simulink model "Trac_Energy_Analysis_Final"  (R2018a)
settings: Solver=VariableStepAuto  StartTime=0.0  StopTime=1220  RelTol=1e-3
libraries: qss_tb_library x2, simulink x1
settings Model: Creator=egp  LastModifiedBy=egp

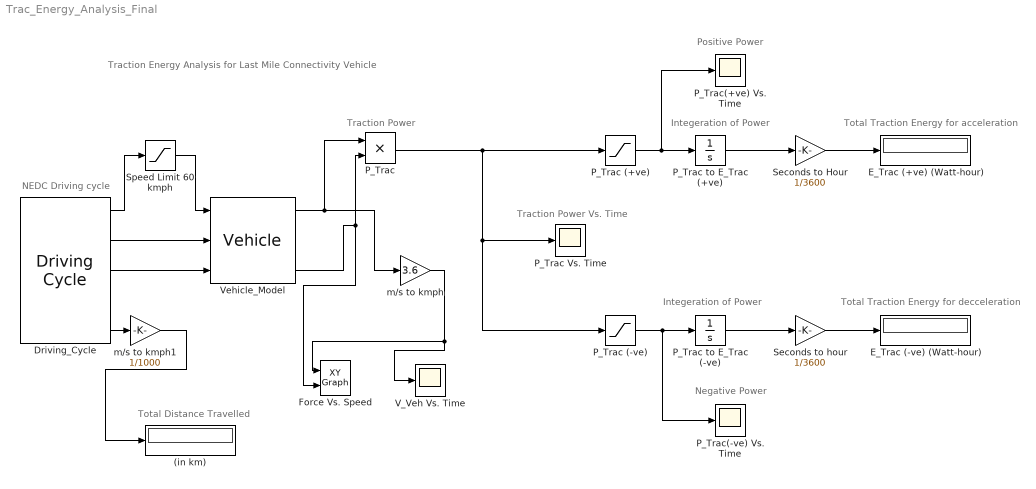
== system Trac_Energy_Analysis_Final ==
  note: Traction Energy Analysis for Last Mile Connectivity Vehicle
  note: Traction Power
  note: NEDC Driving cycle
  note: Total Distance Travelled
  note: Traction Power Vs. Time
  note: Total Traction Energy for acceleration
  note: Total Traction Energy for decceleration
  note: Positive Power
  note: Negative Power
  note: Integeration of Power
  note: Integeration of Power
  (in km) : Display
  Driving_Cycle : qss_tb_library/Driving Cycle/Driving Cycle  Tag=cycle  cyclename1=NEDC  stepsize=1  autostop=on
  E_Trac (+ve) (Watt-hour) : Display
  E_Trac (-ve) (Watt-hour) : Display
  Force Vs. Speed : simulink/Sinks/XY Graph  xmin=0  xmax=65  ymin=-2500  ymax=2500  st=-1
  P_Trac : Product
  P_Trac (+ve) : Saturate  UpperLimit=60000  LowerLimit=0  OutMin=0  OutMax=60000
  P_Trac (-ve) : Saturate  UpperLimit=0  LowerLimit=-60000  OutMin=-60000  OutMax=0
  P_Trac Vs. Time : Scope
  P_Trac to E_Trac (+ve) : Integrator
  P_Trac to E_Trac (-ve) : Integrator
  P_Trac(+ve) Vs. Time : Scope
  P_Trac(-ve) Vs. Time : Scope
  Seconds to Hour : Gain  Gain=1/3600
  Seconds to hour : Gain  Gain=1/3600
  Speed Limit 60 kmph : Saturate  UpperLimit=60/3.6  LowerLimit=0  OutMin=0  OutMax=60/3.6
  V_Veh Vs. Time : Scope
  Vehicle_Model : qss_tb_library/Vehicle/Vehicle  Tag=vehicle  m_f=1750  A_f=2.88  cw=0.5  mu=0.01  k_inertia=5
  m/s to kmph : Gain  Gain=3.6
  m/s to kmph1 : Gain  Gain=1/1000
  wires:
  Driving_Cycle/2 -> Vehicle_Model/2
  Driving_Cycle/3 -> Vehicle_Model/3
  Vehicle_Model/1 -> P_Trac/1, m/s to kmph/1
  Vehicle_Model/3 -> P_Trac/2, Force Vs. Speed/2
  P_Trac/1 -> P_Trac Vs. Time/1, P_Trac (-ve)/1, P_Trac (+ve)/1
  Driving_Cycle/5 -> m/s to kmph1/1
  P_Trac (+ve)/1 -> P_Trac(+ve) Vs. Time/1, P_Trac to E_Trac (+ve)/1
  P_Trac (-ve)/1 -> P_Trac(-ve) Vs. Time/1, P_Trac to E_Trac (-ve)/1
  m/s to kmph/1 -> Force Vs. Speed/1, V_Veh Vs. Time/1
  Driving_Cycle/1 -> Speed Limit 60 kmph/1
  Speed Limit 60 kmph/1 -> Vehicle_Model/1
  P_Trac to E_Trac (+ve)/1 -> Seconds to Hour/1
  Seconds to Hour/1 -> E_Trac (+ve) (Watt-hour)/1
  P_Trac to E_Trac (-ve)/1 -> Seconds to hour/1
  Seconds to hour/1 -> E_Trac (-ve) (Watt-hour)/1
  m/s to kmph1/1 -> (in km)/1
